simulink model "Final_2023_Ejercicio_1_simulink"  (R2016a)
settings: Solver=VariableStepAuto  StartTime=0.0  StopTime=5  RelTol=1e-3
libraries: simulink x1
settings Model: Creator=Abel  LastModifiedBy=Abel

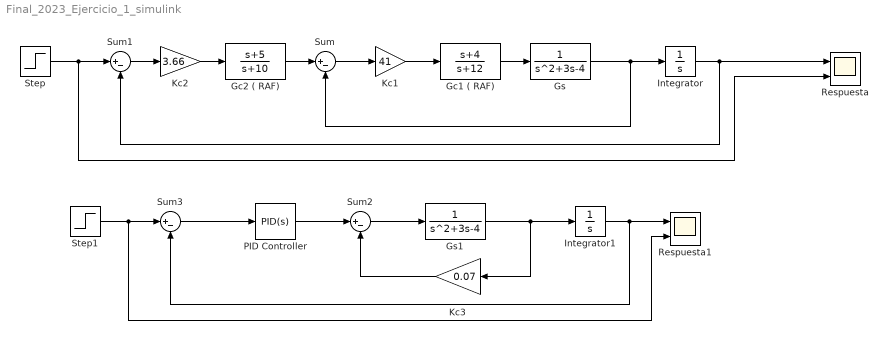
== system Final_2023_Ejercicio_1_simulink ==
  Gc1 ( RAF) : TransferFcn  Numerator=[1 4]  Denominator=[1 12]
  Gc2 ( RAF) : TransferFcn  Numerator=[1 5]  Denominator=[1 10]
  Gs : TransferFcn  Numerator=1  Denominator=[1 3 -4]
  Gs1 : TransferFcn  Numerator=1  Denominator=[1 3 -4]
  Integrator : Integrator
  Integrator1 : Integrator
  Kc1 : Gain  Gain=41
  Kc2 : Gain  Gain=3.66
  Kc3 : Gain  Gain=0.07
  PID Controller : simulink/Continuous/PID Controller  Controller=PID  TimeDomain=Continuous-time  SampleTime=-1  IntegratorMethod=Forward Euler  FilterMethod=Forward Euler  Form=Parallel  UseFilter=on  ControllerParametersSource=internal  P=132.189  I=22.661  D=94.421  N=1  InitialConditionSource=internal  InitialConditionForIntegrator=0  InitialConditionForFilter=0  ExternalReset=none  LimitOutput=off  UpperSaturationLimit=inf  LowerSaturationLimit=-inf  LinearizeAsGain=on  AntiWindupMode=none  Kb=1  TrackingMode=off  Kt=1  PParamMin=[]  PParamMax=[]  IParamMin=[]  IParamMax=[]  DParamMin=[]  DParamMax=[]  NParamMin=[]  NParamMax=[]  KbParamMin=[]  KbParamMax=[]  KtParamMin=[]  KtParamMax=[]  POutMin=[]  POutMax=[]  IOutMin=[]  IOutMax=[]  DOutMin=[]  DOutMax=[]  NOutMin=[]  NOutMax=[]  KbOutMin=[]  KbOutMax=[]  KtOutMin=[]  KtOutMax=[]  IntegratorOutMin=[]  IntegratorOutMax=[]  FilterOutMin=[]  FilterOutMax=[]  SumOutMin=[]  SumOutMax=[]  SumI1OutMin=[]  SumI1OutMax=[]  SumI2OutMin=[]  SumI2OutMax=[]  SumI3OutMin=[]  SumI3OutMax=[]  SumDOutMin=[]  SumDOutMax=[]  SaturationOutMin=[]  SaturationOutMax=[]  IntegratorContinuousStateAttributes=''  IntegratorStateMustResolveToSignalObject=off  IntegratorRTWStateStorageClass=Auto  FilterContinuousStateAttributes=''  FilterStateMustResolveToSignalObject=off  FilterRTWStateStorageClass=Auto  DifferentiatorICPrevScaledInput=0  DifferentiatorOutMin=[]  DifferentiatorOutMax=[]
  Respuesta : Scope  NumInputPorts=2
  Respuesta1 : Scope  NumInputPorts=2
  Step : Step  Time=0  SampleTime=0
  Step1 : Step  Time=0  SampleTime=0
  Sum{,1..3} (4 alike) : Sum  Inputs=|+-
  wires:
  Gs/1 -> Sum/2, Integrator/1
  Integrator/1 -> Respuesta/1, Sum1/2
  Step/1 -> Respuesta/2, Sum1/1
  Sum1/1 -> Kc2/1
  Gc2 ( RAF)/1 -> Sum/1
  Kc2/1 -> Gc2 ( RAF)/1
  Gc1 ( RAF)/1 -> Gs/1
  Kc1/1 -> Gc1 ( RAF)/1
  Sum/1 -> Kc1/1
  Gs1/1 -> Kc3/1, Integrator1/1
  Integrator1/1 -> Respuesta1/1, Sum3/2
  Step1/1 -> Respuesta1/2, Sum3/1
  Sum3/1 -> PID Controller/1
  PID Controller/1 -> Sum2/1
  Sum2/1 -> Gs1/1
  Kc3/1 -> Sum2/2
